simulink model "qless_forgetting_factor_16x16"  (R2021a)
settings: Solver=FixedStepDiscrete  StartTime=0.0  StopTime=stoptime*inf  RelTol=1e-3
InitFcn:
  | qless_init_16chan_fi
undefined symbols (not defined in the file): fc, numArrayElements, physconst, srcAngles, sv, Ts
libraries: hdlsllib x137, commfilt2 x4, commrfcorlib x3, commsync2 x3, commrflib2 x2, commrandsrc3 x2, phasedtxrxlib x2, commdigbbndcpm2 x1, simulink x1, embreciprocals x1, commdigbbndpm3 x1
(part 20 of 22)

== matlab function qless_forgetting_factor_16x16/MVDR_QLess_HDL/Complex Partial-Systolic Matrix Solve Using Q-less QR Decomposition with Forgetting Factor Manually Tiled n=16/Complex Q-less QR Forward Backward Substitute/Complex Burst Back Substitute with Matrix Output1/Reciprocal of the diagonal element/Select diagonal element ==
  data: rIn input; y output; start input; validIn input; validOut output; n parameter
function [y, validOut] = selectDiagonalElement(rIn, start, validIn, n)
%selectDiagonalElement Select diagonal element
%   [y, validOut] = selectDiagonalElement(rIn, start, validIn, m, n)
%   selects a diagonal element from a row of the R matrix, the inverse of
%   which is used in the back substitute computation.
%
%   See also fixed.internal.matrixsolve.selectDiagonalElement.
%
%   Copyright 2019 The MathWorks, Inc.
    
%#codegen

%% INPUTS
% 'rIn' - A non-zero row of the R matrix from the QR decomposition.
%
% 'start' - A boolean signal indicating that a new backsubstitute has
% begun; it thus indicates that new data should be expected.
%
% 'validIn' - A boolean signal indicating that the data on the 'rRow' input
% line is valid.
%
% 'n' (parameter) - The number of columns in the A matrix (and thus rows
% in the R matrix).

%% OUTPUTS
% 'y' - The diagonal element that needs to be inverted.
%
% 'validOut' - A boolean signal indicating that the data on the 'y' output
% line is valid.

%% PERSISTENTS
% 'i' - Counter, and thus tracks which element of the given row needs to be
% inverted. It it initialized to 'numRows' and counts backwards.
%
% 'started' - Indicates if a computation has begun.
persistent i started;

%% CONSTANTS
% 'initialValue', 'finalValue', 'incr' - Constants that help us control the
% behavior of the state machine that selects diagonal elements. If
% 'initialValue' is less than 'finalValue', then the machine is expected to
% perform forward-substitution, and 'incr' should be set to 1. If
% vice-versa, then back-substitution will be performed and 'incr' should be
% set to -1.
initialValue = int16(coder.const(n));
finalValue   = int16(coder.const(1));
incr         = int16(coder.const(-1));

%% MAIN LOOP
if isempty(i)
    % Default persistents. 
    i        = initialValue;
    started  = false;
end

[y,...              % Outputs
 validOut,...
 i,...              % Persistents
 started] = ...  
 fixed.internal.matrixsolve.selectDiagonalElement(rIn,...          % Inputs
                                                  start,...
                                                  validIn,...
                                                  initialValue,... % Constants
                                                  finalValue,...
                                                  incr,...
                                                  i,...            % Persistents 
                                                  started);                       

end

== matlab function qless_forgetting_factor_16x16/MVDR_QLess_HDL/Complex Partial-Systolic Matrix Solve Using Q-less QR Decomposition with Forgetting Factor Manually Tiled n=16/Complex Q-less QR Forward Backward Substitute/Complex Burst Forward Substitute with Matrix Output/Forward substitute logic/Forward substitute state machine ==
  settings: fimath=hdlfimath
  data: rowToSubtract1 output size=[1 p]; rowToSubtract2 output size=[1 p]; inverseElement input size=1; inverseShift input size=1; rIn input size=[1 n]; cIn input size=[1 p]; validIn input boolean size=1; start input boolean size=1; restart input boolean size=1; subtractedRow input size=[1 p]; addedRow input size=[1 p]; multipliedRow input size=[1 p]; finalMultipliedRow input size=[1 p]; rowToAdd1 output size=[1 p]; rowToAdd2 output size=[1 p]; rowToMultiply output size=[1 p]; rElement output size=1; finalRowToMultiply output size=[1 p]; reciprocal output size=1; shiftValue output size=1; xMatrix output size=[n p]; ready output boolean size=1; rowReady output boolean size=1; validOut output boolean size=1; n parameter size=1; p parameter size=1
function [rowToSubtract1,...
          rowToSubtract2,...
          rowToAdd1,...
          rowToAdd2,...
          rowToMultiply,...
          rElement,...
          finalRowToMultiply,...
          reciprocal,...
          shiftValue,...
          xMatrix,...
          ready,...
          rowReady,...
          validOut] = forwardsubStateMachine(inverseElement,...
                                          inverseShift,...
                                          rIn,...
                                          cIn,...
                                          validIn,...
                                          start,...
                                          restart,...
                                          subtractedRow,...
                                          addedRow,...
                                          multipliedRow,...
                                          finalMultipliedRow,...
                                          n,...
                                          p)
%forwardsubStateMachine Implements a state machine that manages the back
%substitute computation to compute the output matrix.
%
%   See also fixed.internal.matrixsolve.selectDiagonalElement.
%
%   Copyright 2019 The MathWorks, Inc.
%#codegen

%% INPUTS
% 'inverseElement' - The reciprocal of the diagonal element to be used
% later.
%
% 'inverseShift' - The reciprocal of the diagonal element is normalized,
% and needs to be denormalized later to yield the correct value.
%
% 'rIn' - A non-zero row of the R matrix from the QR decomposition.
%
% 'cIn' - A row of the Q'B matrix, where Q is obtained from the QR
% decomposition.
%
% 'validIn' - A boolean signal indicating that the data on the input lines
% is valid.
%
% 'start' - A boolean signal indicating that a new backsubstitute has
% begun; it thus indicates that new data should be expected.
%
% 'restart' - A boolean signal to reset the internal state of the block if
% necessary.
%
% 'subtractedRow' - The result of the subraction of the accumulated
% products of the non-diagonal elements of the supplied 'rIn' with the
% rows of the solution matrix, from 'cIn'.
%
% 'addedRow' - The accumulation of the products of the non-diagonal
% elements of the supplied 'rIn' with the rows of the solution matrix.
%
% 'multipliedRow' - The product of a non-diagonal element of the supplied
% 'rIn' with a row from the solution matrix.
%
% 'finalMultipliedRow' - The multiplication of the 'subractedRow' with the
% 'inverseElement' - after shifting by 'inverseShift', this is thus a row
% of the solution matrix.
%
% 'm' (parameter) - The number of rows in A and B matrices.
%
% 'n' (parameter) - The number of columns in the A matrix (and thus rows
% in the R matrix).
%
% 'p' (parameter) - The number of columns in the B matrix (and thus columns
% in the R matrix).

%% OUTPUTS
% 'rowToSubtract1' - This is essentially 'cIn'; we want to subtract the
% accumulated sum (of the products of the non-diagonal elements of 'rIn'
% with the rows of the solution matrix).
%
% 'rowToSubtract2' - This is the accumulated sum of the products of the
%  non-diagonal elements of 'rIn' with the rows of the solution matrix.
%
% 'rowToAdd1' - This is the accumulated sum, so far, of the products of the
%  non-diagonal elements of 'rIn' with the rows of the solution matrix.
%
% 'rowToAdd2' - This is 'multipliedRow' - the product of a non-diagonal
% element of 'rIn' with a row of the solution matrix.
%
% 'rowToMultiply' - A row of the solution matrix - same as 'previousRow'.

% 'rElement' - A non-diagonal element of the supplied 'rIn', to be used to
% multiply with a row of the solution matrix.
%
% 'finalRowToMultiply' - The result of the subraction of the accumulated
% products of the non-diagonal elements of the supplied 'rIn' with the
% rows of the solution matrix, from 'cIn'.
%
% 'reciprocal' - The reciprocal of the diagonal element - same as
% 'inverseElement'.
%
% 'shiftValue' - An integer value used to denormalize the reciprocal - same
% as 'inverseShift'.
%
% 'xMatrix' - The solution to A\B.
%
% 'ready' - A boolean signal indicating the end of computation for the
% entire backsubstitute; it goes high AFTER all the rows of the solution
% matrix have been streamed out.
%
% 'rowReady' - A boolean signal indicating (to the connected logic in the
% hierarchy) that a row of the solution matrix has been computed, and thus
% to signal that the block is ready to accept new data.
%
% 'validOut' - A boolean signal indicating that the data on the output line
% 'outputRow' is valid.

%% PERSISTENTS
% 'mState' - An integer value to hold the state for this FSM. Full
% specifics are listed as comments for each case for this variable.
%
% 'rowCounter' - An integer tracking the row of the solution matrix we are
% currently working on.
%
% 'iterCounter' - An integer tracking which rows of the solution matrix
% have been fetched from the RAM already.
%
% 'sumOfProducts' - The accumulated sum of the products of the non-diagonal
% elements of the supplied 'rIn' with the rows of the solution matrix.
%
% 'finalRowInternal' - Same as finalMultipliedRow.
%
% 'outputMatrix' - The solution to A\B.
%
% 'ramCycleCounter' - An integer counter to track how many cycles have
% passed by since a row of the solution matrix was requested from the RAM.
%
% 'realComplexCycleCounter' - An integer counter to track how many cycles
% have passed by since a real number was multiplied with a complex vector.
%
% 'complexComplexCycleCounter' - An integer counter to track how many
% cycles have passed by since a complex number was multiplied with a
% complex vector.
persistent mState;
persistent rowCounter;
persistent iterCounter;
persistent sumOfProducts;
persistent finalRowInternal;
persistent outputMatrix;
persistent ramCycleCounter;
persistent realComplexCycleCounter;
persistent complexComplexCycleCounter;

%% Get Constants
isComplex = false;
[defaultState,...
    numRows,...
    numColsB,...
    numRamCycles,...
    numRealComplexMulCycles,...
    numComplexComplexMulCycles] = fixed.internal.matrixsolve.getBacksubStateConstants(n,p,isComplex);

%% MAIN LOOP
if isempty(mState)
    % Default persistents.
    mState                      = defaultState;
    rowCounter                  = numRows;
    iterCounter                 = numRows;
    sumOfProducts               = zeros(1, numColsB, 'like', cIn);
    finalRowInternal            = zeros(1, numColsB, 'like', cIn);
    outputMatrix                = zeros(n, p, 'like', cIn);
    ramCycleCounter             = numRamCycles;
    realComplexCycleCounter     = numRealComplexMulCycles;
    complexComplexCycleCounter  = numComplexComplexMulCycles;
end

% [rowToSubtract1,... % Outputs
%  rowToSubtract2,...
%  rowToAdd1,...
%  rowToAdd2,...
%  rowToMultiply,...
%  rElement,...
%  finalRowToMultiply,...
%  reciprocal,...
%  shiftValue,...
%  xMatrix,...
%  ready,...
%  rowReady,...
%  validOut,...
%  mState,...          % Persistents
%  rowCounter,...
%  iterCounter,...
%  sumOfProducts,...
%  finalRowInternal,...
%  ramCycleCounter,...
%  realComplexCycleCounter,...
%  complexComplexCycleCounter] = ...
%  fixed.internal.matrixsolve.forwardsubStateMachineStreamOutMatrix( inverseElement,...  % Inputs
%                                                                 inverseShift,...
%                                                                 rIn,...
%                                                                 cIn,...
%                                                                 validIn,...
%                                                                 start,...
%                                                                 subtractedRow,...
%                                                                 addedRow,...
%                                                                 multipliedRow,...
%                                                                 finalMultipliedRow,...
%                                                                 restart,...
%                                                                 numRows,...         % Constants 
%                                                                 numColsB,...                  
%                                                                 numRamCycles,...                
%                                                                 numRealComplexMulCycles,...
%                                                                 numComplexComplexMulCycles,...
%                                                                 mState,...          % Persistents
%                                                                 rowCounter,...
%                                                                 iterCounter,...
%                                                                 sumOfProducts,...
%                                                                 finalRowInternal,...
%                                                                 outputMatrix,...
%                                                                 ramCycleCounter,...
%                                                                 realComplexCycleCounter,...
%                                                                 complexComplexCycleCounter);

% Describe all possible states.
numStates                   = coder.const(uint8(10));
statesNT                    = numerictype(0, nextpow2(numStates), 0);
defaultState                = fi(0, statesNT);
waitForValidInState         = fi(1, statesNT);
waitForFinalAnswerState     = fi(2, statesNT);
waitForMultiplicationState  = fi(3, statesNT);
waitForAdditionState        = fi(4, statesNT);
waitForSubtractionState     = fi(7, statesNT);

% MAIN LOOP
% NOTE: 'cIn' has the same type as 'previousRow', so they can be used
% interchangeably.

% Default outputs.
rowToSubtract1              = cIn;
rowToSubtract2              = zeros(1, numColsB, 'like', cIn);
rowToAdd1                   = zeros(1, numColsB, 'like', cIn);
rowToAdd2                   = zeros(1, numColsB, 'like', cIn);
rowToMultiply               = zeros(1, numColsB, 'like', cIn);
rElement                    = cast(1, 'like', rIn);
finalRowToMultiply          = cIn;
reciprocal                  = inverseElement;
shiftValue                  = int32(0);
xMatrix                     = zeros(numRows, numColsB, 'like', cIn);
ready                       = false;
rowReady                    = false;
validOut                    = false;

if restart
     % Default persistents.
     isComplex = coder.const(any(~isreal(cIn)));
    [mState,...
    rowCounter,...
    iterCounter,...
    sumOfProducts,...
    finalRowInternal,...
    ramCycleCounter,...
    realComplexCycleCounter,...
    complexComplexCycleCounter] = fixed.internal.matrixsolve.setDefaultPersistentVars(numRows, numColsB, isComplex, cIn);
    outputMatrix = zeros(numRows, numColsB, 'like', cIn);
else
    switch mState
        % STATE 0 - Default case - we end up here at the beginning and
        % the end of each computation, never in between. Wait for 'start'
        % and validIn to go high.
        case defaultState
            % If both 'start' and 'validIn' are high, go to state 2
            % directly and wait for 'finalMultipliedRow'.
            if start && validIn
                rowCounter = numRows;
                mState     = waitForFinalAnswerState;
                % Otherwise, go to state 1 and wait for 'validIn'.
            elseif start
                mState     = waitForValidInState;
                ready      = true;
                % Otherwise, stay here and wait for 'start'/'validIn'.
            else
                mState     = defaultState;
                ready      = true;
            end
            
            % STATE 1 - Wait for 'validIn', but also move to other states
            % depending on some internal variables.
        case waitForValidInState
            % How many iterations do we need?
            iterCounter = numRows;
            
            % Are we done already? Check 'rowCounter' to find out; if yes,
            % stream out the matrix and move to default state.
            if isequal(rowCounter, 0)
                mState          = defaultState;
                ready           = true;
                validOut        = true;
                xMatrix         = outputMatrix;
                rowCounter(:)   = numRows;
                % If this is the first row (from the bottom), then move to
                % state 2 to wait for the final row.
            elseif validIn && isequal(rowCounter, numRows)
                mState          = waitForFinalAnswerState;
                % If not, then multiply previous row with last element of
                % 'rIn'. Then go to state 3, which is the dedicated
                % multiplication state
            elseif validIn
                rowToMultiply   = outputMatrix(numRows, :);
                rElement        = rIn(1);
                mState          = waitForMultiplicationState;
            else
                mState(:)       = waitForValidInState;
            end
            
            % STATE 2 - Wait for 'finalMultipliedRow'.
        case waitForFinalAnswerState
            shiftValue(:)                   = inverseShift;
            finalRowToMultiply              = finalRowInternal;
            % If we get the data on this cycle...
            if isequal(realComplexCycleCounter, 1)
                outputMatrix(rowCounter, :) = finalMultipliedRow;
                % Give values to persistent variables for the next cycle, and set
                % 'rowReady' to high.
                rowReady                    = true;
                mState                      = waitForValidInState;
                realComplexCycleCounter     = numRealComplexMulCycles;
                rowCounter(:)               = rowCounter - 1;
                % ...otherwise, wait here.
            else
                realComplexCycleCounter(:)  = realComplexCycleCounter - 1;
            end
            
            % STATE 3 - Wait for 'multipliedRow'.
        case waitForMultiplicationState
            shiftValue(:)                     = 0;
            % If we get the data on this cycle...
            if isequal(complexComplexCycleCounter, 1)
                % Add the new 'multipliedRow' to the accumulated sum of
                % products so far, and move to state 4.
                rowToAdd1                     = sumOfProducts;
                rowToAdd2                     = multipliedRow;
                mState                        = waitForAdditionState;
                iterCounter(:)                = iterCounter - 1;
                complexComplexCycleCounter    = numComplexComplexMulCycles;
                % ...otherwise, wait here.
            else
                complexComplexCycleCounter(:) = complexComplexCycleCounter - 1;
            end
            
            % STATE 4 - Wait for 'addedRow'. Since addition only takes a single
            % cycle, when we get here we should already have the addition.
        case waitForAdditionState
            sumOfProducts       = addedRow;
            % Now do we go back and do more multiplications, or do we go to
            % subtract the accumulated sum from 'cIn'?
            if isequal(iterCounter, rowCounter)
                rowToSubtract1  = cIn;
                rowToSubtract2  = addedRow;
                mState          = waitForSubtractionState;
            else
                % If iterations are left, fetch more data from the RAM.
                rowToMultiply   = outputMatrix(iterCounter, :);
                rElement        = rIn(numRows + 1 - iterCounter);
                mState          = waitForMultiplicationState;
            end
            
            % STATE 7 - Wait for 'subtractedRow'. Since subtraction only takes
            % a single cycle, when we get here we should already have the
            % subtraction. Then move to state 2 to get 'finalMultipliedRow'.
        case waitForSubtractionState
            reciprocal          = inverseElement;
            finalRowToMultiply  = subtractedRow;
            mState              = waitForFinalAnswerState;
            sumOfProducts       = zeros(1, numColsB, 'like', cIn);
            finalRowInternal    = subtractedRow;
            
            % Catch all other states and go to the default state. Also set all
            % persistent variables to their default values.
        otherwise
            mState                      = defaultState;
            rowCounter                  = numRows;
            iterCounter                 = numRows;
            sumOfProducts               = zeros(1, numColsB, 'like', cIn);
            finalRowInternal            = zeros(1, numColsB, 'like', cIn);
            ramCycleCounter             = numRamCycles;
            realComplexCycleCounter     = numRealComplexMulCycles;
            complexComplexCycleCounter  = numComplexComplexMulCycles;
    end
end


end

== matlab function qless_forgetting_factor_16x16/MVDR_QLess_HDL/Complex Partial-Systolic Matrix Solve Using Q-less QR Decomposition with Forgetting Factor Manually Tiled n=16/Complex Q-less QR Forward Backward Substitute/Complex Burst Forward Substitute with Matrix Output/Forward substitute logic/Variable shift/MATLAB Function ==
  settings: fimath=hdlfimath
  data: x input size=[1 p]; y output size=[1 p]; shiftValue input
function y = fcn(x,shiftValue)
    if isfi(x) && isscaledtype(x)
        y = bitshift(x, shiftValue);
    else
        y = cast(double(x)* 2.^double(shiftValue),'like',x);
    end
end

== matlab function qless_forgetting_factor_16x16/MVDR_QLess_HDL/Complex Partial-Systolic Matrix Solve Using Q-less QR Decomposition with Forgetting Factor Manually Tiled n=16/Complex Q-less QR Forward Backward Substitute/Complex Burst Forward Substitute with Matrix Output/Cast to Union of Types ==
  settings: fimath=hdlfimath
  data: Xref input; Cout output; Cin input
function Cout = castToUnionType(Xref,Cin)
    %castToUnionType Cast second input to union of the two types
    T = fixed.internal.type.unionPrototype(Cin,Xref,...
        'RoundingMethod','Floor',...
        'OverflowAction','Wrap');
    Cout = cast(Cin,'like',T);
end

== matlab function qless_forgetting_factor_16x16/MVDR_QLess_HDL/Complex Partial-Systolic Matrix Solve Using Q-less QR Decomposition with Forgetting Factor Manually Tiled n=16/Complex Q-less QR Forward Backward Substitute/Complex Burst Forward Substitute with Matrix Output/Reciprocal of the diagonal element/Positive Normalized Reciprocal HDL Optimized/Positive Real CORDIC Reciprocal Kernel HDL Optimized/positiveNormalizedCORDICReciprocal ==
  settings: fimath=hdlfimath
  data: x input; t_in input; y output; t output; validIn input; validOut output
function [y, t, validOut] = positiveNormalizedCORDICReciprocal(x, t_in, validIn)
%positiveNormalizedCORDICReciprocal Positive normalized reciprocal
%   [y, t, validOut] = positiveNormalizedCORDICReciprocal(x, t_in, validIn)
%   produces y = 1/x when 1 <= x < 2, and t = t_in.
%
%   When x = 0 and x is fixed-point or scaled-double, then y = 2 - eps(y).
%
%   When x = 0 and x is a floating-point type, then y = inf.
%
%   If x is fixed-point, then y is fixed-point with
%   numerictype(1, x.WordLength, x.WordLength - 2).
%
%   If x is floating-point, then y is floating-point of the same type.
%
%   References:
%
%   [1] Jack E. Volder, "The CORDIC Trigonometric Computing Technique," IRE
%       Transactions on Electronic Computers, Volume EC-8, September 1959,
%       pp. 330-334.
%
%   [2] J.S. Walther, "A Unified Algorithm for Elementary Functions,"
%       Conference Proceedings, Spring Joint Computer Conference, May 1971,
%       pp. 379-385.
%
%   See also fixed.internal.reciprocal.cordicReciprocalKernel.

%   Copyright 2019 The MathWorks, Inc.
%#codegen
    fixed.internal.reciprocal.validateReciprocalInputs(x, validIn);
    if isfi(x) && isscaledtype(x)
        % CORDIC reciprocal for fixed-point and scaled-double types
        [y,t,validOut] = fixedpointReciprocal(x,t_in,validIn);
    else
        % y = 1/x for builtin types.
        y = 1./x;
        t = t_in;
        validOut = validIn;
    end
end

function [reciprocal, t, validOut] = fixedpointReciprocal(xIn,t_in, validIn)
%fixedpointReciprocal Fixed-point reciprocal
%   [reciprocal, t, validOut] = fixedpointReciprocal(xIn, t_in, validIn)
%   Given real scalar xIn such that 1 <= xIn < 2 this function produces
%   reciprocal such that
%
%      reciprocal = 1/xIn.
%
%   and reciprocal is in the range 0.5 < reciprocal <= 1.
%
%   When xIn = 0, then y = 2 - eps(y).
%
%   The input is only valid when validIn = true.  The output is only
%   valid when validOut = true.
%
%   The output t is identical to t_in, synchronized by validIn/validOut.
    [T,NumberOfCordicIterations] = fixed.internal.reciprocal.positiveReciprocalTypes(xIn);
    % Register variables for the CORDIC Reciprocal Kernel
    persistent xReg yReg zReg validReg tReg
    if isempty(xReg)
        xReg = zeros(NumberOfCordicIterations+2,1,'like',T.x);
        yReg = zeros(NumberOfCordicIterations+2,1,'like',T.x);
        zReg = zeros(NumberOfCordicIterations+2,1,'like',T.x);
        validReg = zeros(NumberOfCordicIterations+2,1,'like',validIn);
        tReg = zeros(NumberOfCordicIterations+2,1,'like',t_in);
    end
    % CORDIC Reciprocal Kernel
    [reciprocal,t,validOut,...
        xReg,yReg,zReg,validReg,tReg... % Persistent variables
        ] = fixed.internal.reciprocal.cordicReciprocalKernel(xIn,t_in,validIn,...
        xReg,yReg,zReg,validReg,tReg... % Persistent variables
        );
end

== matlab function qless_forgetting_factor_16x16/MVDR_QLess_HDL/MATLAB Function ==
  data: write_en output; valid_i input; isEmpty input; qr_ready input; read_en output
function [write_en, read_en]= amat_scheduler(valid_i, isEmpty, qr_ready)
persistent scheduler_state counter

STATE_IS_LOADING_MAT = fi(0,0,4,0);
WAIT_FOR_SOLVE = fi(1,0,4,0);
MAX_FIFO_DEPTH = 16;
if isempty(scheduler_state)
    scheduler_state = STATE_IS_LOADING_MAT;
    counter = uint32(0);
end

write_en = false;
read_en = false;
switch(scheduler_state)
    case(STATE_IS_LOADING_MAT)
        if valid_i
            if counter < MAX_FIFO_DEPTH
                write_en = true;
                counter(:) = counter + 1;
            else
                scheduler_state(:) = WAIT_FOR_SOLVE;
                counter(:) = 0;            
            end            
        end
    case(WAIT_FOR_SOLVE)
        if qr_ready
            if counter < MAX_FIFO_DEPTH
                read_en = true;
                counter(:) = counter + 1; 
            else
                scheduler_state(:) = STATE_IS_LOADING_MAT;
                counter(:) = 0;         
            end
        end
       
end



%  if isEmpty
%             scheduler_state(:) = STATE_IS_LOADING_MAT;
%         else
%             if qr_ready
%                 read_en = true;
%             end
%  end
%         
 
% if ~isEmpty && qr_ready
%     read_en = true;
% end


end

== matlab function qless_forgetting_factor_16x16/MVDR_QLess_HDL/Complex Partial-Systolic Matrix Solve Using Q-less QR Decomposition with Forgetting Factor Manually Tiled n=16/Complex Q-less QR Forward Backward Substitute/Complex Burst Forward Substitute with Matrix Output/Reciprocal of the diagonal element/Positive Normalized Reciprocal HDL Optimized/Positive Real Normalizer HDL Optimized/positiveRealNormalizer ==
  settings: fimath=hdlfimath
  data: u input; x output; validIn input; e output; validOut output
function [x, e, validOut] = positiveRealNormalizer(u, validIn)
%positiveRealNormalizer  Positive real normalizer
%   [x, e, validOut] = positiveRealNormalizer(u, validIn) produces
%   x such that 1 <= x < 2 and e such that x = (2^e)*u when u > 0.
%
%   When u = 0 and u is fixed-point or scaled-double, then x = 0 and
%   e = (2^nextpow2(x.WordLength)) - x.WordLength - x.FractionLength.
%
%   When u = 0 and u is floating-point, then x = 0 and e = 1.
%
%   See also fixed.internal.reciprocal.normalizePositiveFixedPoint,
%   fixed.internal.reciprocal.normalizePositiveFloatOrScaledDouble.

%   Copyright 2019 The MathWorks, Inc.
%#codegen

% This function only works on scalars.
% Only operate on the real part
    fixed.internal.reciprocal.validateNormalizerInputs(u, validIn);
    % Normalize in unsigned type.
    [x_normalized, n_normalized, validOut] = normalize(real(u), validIn);
    % Cast the output to signed if the input was signed.
    x = fixed.internal.reciprocal.castToInputSignedness(x_normalized,u);
    % Convert the normalized shift value based on the data type of the
    % input U so that the output of the normalizer X is in real-world
    % scale and X = (2^N)*U.
    e = fi(int32(0));
    e(:) = fixed.internal.reciprocal.normalizedShiftToRealWorldValueShift(n_normalized,u);
end

function [x_normalized, e_normalized, validOut] = normalize(u, validIn)
    if isfi(u) && isfixed(u)
        % Normalize fixed-point values
        [x_normalized, e_normalized,validOut] = normalizeFixedpoint(u, validIn);
    else
        % Normalize floating-point or scaled-double
        [x_normalized, e_normalized, validOut] = fixed.internal.reciprocal.normalizePositiveFloatOrScaledDouble(u, validIn);
    end
end

function [u_normalized, e_normalized,validOut] = normalizeFixedpoint(u, validIn)
% Normalize fixed-point values.
    persistent validReg
    persistent tReg
    persistent xReg
    % For fixed-point types, the normalization uses a binary search of
    % length log2 of the word length of the input.
    number_of_stages = coder.const(nextpow2(u.WordLength));

    if isempty(validReg)
        validReg = false(number_of_stages+1,1);
        tReg = zeros(number_of_stages+1,1,'like',fi(0,0,max(number_of_stages,1),0));
        xReg = zeros(number_of_stages+1,1,'like',fi([],0,u.WordLength,0));
    end

    [u_normalized, e_normalized,validOut,...
        validReg, tReg,xReg...  % Persistent
        ] = fixed.internal.reciprocal.normalizePositiveFixedPoint(u, validIn, number_of_stages, ...
        validReg, tReg,xReg...  % Persistent
        );
end

== matlab function qless_forgetting_factor_16x16/MVDR_QLess_HDL/Complex Partial-Systolic Matrix Solve Using Q-less QR Decomposition with Forgetting Factor Manually Tiled n=16/Complex Q-less QR Forward Backward Substitute/Complex Burst Forward Substitute with Matrix Output/Reciprocal of the diagonal element/Select diagonal element ==
  data: rIn input; y output; start input; validIn input; validOut output; n parameter
function [y, validOut] = selectDiagonalElement(rIn, start, validIn, n)
%selectDiagonalElement Select diagonal element
%   [y, validOut] = selectDiagonalElement(rIn, start, validIn, m, n)
%   selects a diagonal element from a row of the R matrix, the inverse of
%   which is used in the back substitute computation.
%
%   See also fixed.internal.matrixsolve.selectDiagonalElement.
%
%   Copyright 2019 The MathWorks, Inc.
    
%#codegen

%% INPUTS
% 'rIn' - A non-zero row of the R matrix from the QR decomposition.
%
% 'start' - A boolean signal indicating that a new backsubstitute has
% begun; it thus indicates that new data should be expected.
%
% 'validIn' - A boolean signal indicating that the data on the 'rRow' input
% line is valid.
%
% 'n' (parameter) - The number of columns in the A matrix (and thus rows
% in the R matrix).

%% OUTPUTS
% 'y' - The diagonal element that needs to be inverted.
%
% 'validOut' - A boolean signal indicating that the data on the 'y' output
% line is valid.

%% PERSISTENTS
% 'i' - Counter, and thus tracks which element of the given row needs to be
% inverted. It it initialized to 'numRows' and counts backwards.
%
% 'started' - Indicates if a computation has begun.
persistent i started;

%% CONSTANTS
% 'initialValue', 'finalValue', 'incr' - Constants that help us control the
% behavior of the state machine that selects diagonal elements. If
% 'initialValue' is less than 'finalValue', then the machine is expected to
% perform forward-substitution, and 'incr' should be set to 1. If
% vice-versa, then back-substitution will be performed and 'incr' should be
% set to -1.
initialValue = int16(coder.const(1));
finalValue   = int16(coder.const(n));
incr         = int16(coder.const(1));

%% MAIN LOOP
if isempty(i)
    % Default persistents. 
    i        = initialValue;
    started  = false;
end

[y,...              % Outputs
 validOut,...
 i,...              % Persistents
 started] = ...  
 fixed.internal.matrixsolve.selectDiagonalElement(rIn,...          % Inputs
                                                  start,...
                                                  validIn,...
                                                  initialValue,... % Constants
                                                  finalValue,...
                                                  incr,...
                                                  i,...            % Persistents 
                                                  started);                       

end

== matlab function qless_forgetting_factor_16x16/MVDR_QLess_HDL/Complex Partial-Systolic Matrix Solve Using Q-less QR Decomposition with Forgetting Factor Manually Tiled n=16/Complex Q-less QR Forward Backward Substitute/Partial-Systolic Matrix Solve Q-less QR B Buffer Manager/B Buffer Manager State Machine ==
  data: rowForFwdSub input; Lrow output; fwdSubValidIn input size=1; bValidIn input size=1; backSubDone input size=1; restart input boolean size=1; rowIndex output fixdt('uint32', 'DataTypeOverride', 'Off') size=1; validOut output boolean size=1; start output boolean size=1; readyForFwdSub output boolean size=1; n parameter size=1
function [Lrow,...
        rowIndex,...
        validOut,...
        start,...
        readyForFwdSub] = ...
        manageBufferForBStateMachine(...
        rowForFwdSub,...
        fwdSubValidIn,...
        bValidIn,...
        backSubDone,...
        restart,...
        n)
    
    % State names
    DEFAULT = uint8(0);
    STARTFORWARDSUBSTITUTE = uint8(1);
    MANAGEFORWARDSUBSTITUTE = uint8(2);
    FINISHFORWARDSUBSTITUTE = uint8(3);
    
    persistent mState
    persistent mRowIndex
    persistent mValidOut
    persistent mStart
    persistent mLrow
    persistent mReadyForFwdSub
    
    % Init persistents.
    if isempty(mState)
        mState = DEFAULT;
        mRowIndex = uint32(1);
        mValidOut = false;
        mStart = false;
        mLrow = zeros(size(rowForFwdSub),'like',rowForFwdSub);
        mReadyForFwdSub = false;
    end
    state = mState;
    rowIndex = mRowIndex;
    validOut = mValidOut;
    start = mStart;
    Lrow = mLrow;
    readyForFwdSub = mReadyForFwdSub;
    if restart
        % If 'restart' is high, re-initialize everything.
        mState = DEFAULT;
        mLrow = rowForFwdSub;
        mRowIndex(:) = 1;
        mValidOut = false;
        mStart = false;
        mReadyForFwdSub = false;
    else
        % Otherwise, enter the main loop.
        mLrow = rowForFwdSub;
        mValidOut = false;
        mStart = false;
        mReadyForFwdSub = false;
        switch state
            case DEFAULT
                % Default state: accept the incoming B matrix when validIn is high,
                % and then move on to the next state.
                if bValidIn
                    mRowIndex(:) = 1;
                    mState(:) = STARTFORWARDSUBSTITUTE;
                    mStart = true;
                    mReadyForFwdSub = true;
                else
                end
                
            case STARTFORWARDSUBSTITUTE
                % Start the forward substitute (i.e., send one
                % row), and then move on to MANAGEFORWARDSUBSTITUTE.
                mReadyForFwdSub = true;
                if fwdSubValidIn
                    mLrow = rowForFwdSub;
                    mValidOut = true;
                    mState(:) = MANAGEFORWARDSUBSTITUTE;
                end
                
            case MANAGEFORWARDSUBSTITUTE
                % Manage the forward substitute. Send a new row from the B
                % matrix when it's needed. At the end, move to
                % FINISHFORWARDSUBSTITUTE.
                if fwdSubValidIn && ~isequal(mRowIndex, n)
                    mRowIndex(:) = mRowIndex + 1;
                    mValidOut = true;
                elseif isequal(mRowIndex, n)
                    mState(:)= FINISHFORWARDSUBSTITUTE;
                else
                end
                
            case FINISHFORWARDSUBSTITUTE
                % Wait for the back substitute to end; then wait to receive
                % another B matrix.
                if backSubDone
                    mState(:) = DEFAULT;
                    mRowIndex(:) = 1;
                end
        end
    end
    
end

== matlab function qless_forgetting_factor_16x16/MVDR_QLess_HDL/Complex Partial-Systolic Matrix Solve Using Q-less QR Decomposition with Forgetting Factor Manually Tiled n=16/Complex Q-less QR Forward Backward Substitute/Partial-Systolic Matrix Solve Q-less QR B Buffer Manager/Save Matrix B/Enabled Delay ==
  data: dataIn input; dataOut output; writeEnable input; restart input
function dataOut = enabledDelay(dataIn,writeEnable,restart)
    persistent mData
    if isempty(mData)
        mData = zeros(size(dataIn),'like',dataIn);
    end
    dataOut = mData;
    if restart
        mData = zeros(size(dataIn),'like',dataIn);
    elseif writeEnable
        mData = dataIn;
    end
end

== matlab function qless_forgetting_factor_16x16/MVDR_QLess_HDL/Complex Partial-Systolic Matrix Solve Using Q-less QR Decomposition with Forgetting Factor Manually Tiled n=16/Complex Q-less QR Forward Backward Substitute/Partial-Systolic Matrix Solve Q-less QR Forward Substitute Memory Manager/MATLAB Function1 ==
  data: rowIndex output fixdt('uint32', 'DataTypeOverride', 'Off') size=1; inputValidIn input; needFwdSubRow input; backSubDone input; restart input; validOut output; needBackSubRow output; n parameter size=1
function [...
        rowIndex,...
        validOut,...
        needBackSubRow] = ...
        fwdSubBuffer(...
        inputValidIn,...
        needFwdSubRow,...
        backSubDone,...
        restart,...
        n)

    % State names
    DEFAULT = uint8(0);
    STARTBACKWARDSUBSTITUTE = uint8(1);
    MANAGEBACKWARDSUBSTITUTE = uint8(2);
    FINISHBACKWARDSUBSTITUTE = uint8(3);

    persistent mRowIndex;
    persistent mState;
    
    % Initialize persistents.
    if isempty(mState)
        mRowIndex = uint32(1);
        mState = DEFAULT;
    end
    
    rowIndex = mRowIndex;
    
    if restart
        % If 'restart' is high, re-initialize everything.
        mRowIndex(:) = 1;
        mState(:) = DEFAULT;
        validOut  = false;
        needBackSubRow = false;
    else
        % Otherwise, enter the main loop.
        validOut  = false;
        needBackSubRow = false;
        switch mState
            case DEFAULT
                % Default state: Accept the output of the forward
                % substitute. Once n rows have been received, move to state
                % STARTFORWARDSUBSTITUTE.
                if inputValidIn
                    mState(:) = STARTBACKWARDSUBSTITUTE;
                    mRowIndex(:) = 1;
                else
                end
                
            case STARTBACKWARDSUBSTITUTE
                % Start the backward substitute (i.e., send a single row)
                % and then move to state MANAGEBACKWARDSUBSTITUTE.
                mRowIndex(:) = 1;
                validOut  = true;
                needBackSubRow = true;
                mState(:) = MANAGEBACKWARDSUBSTITUTE;
                
            case MANAGEBACKWARDSUBSTITUTE
                % Manage the backward substitute. Send a new row from the
                % assembled matrix when it's needed. At the end, move to
                % state FINISHBACKWARDSUBSTITUTE.
                if needFwdSubRow && ~isequal(mRowIndex, n)
                    mRowIndex(:) = mRowIndex + 1;
                    validOut  = true;
                    needBackSubRow = true;
                elseif isequal(mRowIndex, n)
                    mState(:) = FINISHBACKWARDSUBSTITUTE;
                else
                end
                
            case FINISHBACKWARDSUBSTITUTE
                % Wait for the backward substitute to end; then move on to
                % the default state.
                if backSubDone
                    mState(:) = DEFAULT;
                    mRowIndex(:) = 1;
                end
        end
    end
end

== matlab function qless_forgetting_factor_16x16/MVDR_QLess_HDL/Complex Partial-Systolic Matrix Solve Using Q-less QR Decomposition with Forgetting Factor Manually Tiled n=16/Complex Q-less QR Forward Backward Substitute/Partial-Systolic Matrix Solve Q-less QR Forward Substitute Memory Manager/Save Matrix B/Enabled Delay ==
  data: dataIn input; dataOut output; writeEnable input; restart input
function dataOut = enabledDelay(dataIn,writeEnable,restart)
    persistent mData
    if isempty(mData)
        mData = zeros(size(dataIn),'like',dataIn);
    end
    dataOut = mData;
    if restart
        mData = zeros(size(dataIn),'like',dataIn);
    elseif writeEnable
        mData = dataIn;
    end
end

== matlab function qless_forgetting_factor_16x16/MVDR_QLess_HDL/Complex Partial-Systolic Matrix Solve Using Q-less QR Decomposition with Forgetting Factor Manually Tiled n=16/Complex Q-less QR Forward Backward Substitute/Partial-Systolic Matrix Solve Q-less QR Output Manager/Partial-Systolic Manage QR Output State Machine ==
  data: validIn input size=1; columnOutIndex output fixdt('uint32', 'DataTypeOverride', 'Off') size=1; needRowFwdSub input size=1; needRowBackSub input size=1; backSubDone input size=1; restartIn input size=1; readyForFwdSub input size=1; fwdSubValidOut output size=1; rowOutIndex output fixdt('uint32', 'DataTypeOverride', 'Off') size=1; n parameter size=1; validR output size=1; restartOut output size=1
function [columnOutIndex,...
        fwdSubValidOut,...
        rowOutIndex,...
        validR,...
        restartOut] = manageQlessOutput(...
        validIn,...
        needRowFwdSub,...
        needRowBackSub,...
        backSubDone,...
        restartIn,...
        readyForFwdSub,...
        n)
    
    % State names
    DEFAULT = uint8(0);
    START = uint8(7);
    FORWARDSUBSTITUTE = uint8(1);
    STARTBACKWARDSUBSTITUTE = uint8(2);
    BACKWARDSUBSTITUTE = uint8(3);
    ENDBACKWARDSUBSTITUTE = uint8(4);
    WAITFORBMATRIX = uint8(5);
    CONTINUEFORWARDSUBSTITUTE = uint8(8);
    BMATRIXREADY = uint8(6);
    
    % Initial output values
    columnOutIndex = uint32(1);
    fwdSubValidOut = false;
    rowOutIndex = uint32(1);
    validR = false;
    restartOut = false;
    
    % persistent r;
    persistent i;
    persistent mState;
    
    % Init persistents.
    if isempty(mState)
        i              = uint32(n);
        mState         = DEFAULT;
    end
    
    
    % If 'restart' is high, re-initialize everything.
    if restartIn
        restartOut = true;
        rowOutIndex(:) = n;
        columnOutIndex(:) = n;
        i(:)           = n;
        mState(:)      = DEFAULT;
    else
        % Otherwise, enter the main loop.
        rowOutIndex(:) = i;
        columnOutIndex(:) = i;
        switch mState
            % Default state: Wait for validIn (the validOut of the previous
            % block) to go high 'n' times, where 'n' is the number of columns
            % in the A matrix. Once validIn goes high 'n' times, 'start' the
            % forward substitution process and move to state FORWARDSUBSTITUTE.
            case DEFAULT
                if validIn
                    validR = true;
                    mState(:) = START;
                    fwdSubValidOut = false;
                    i(:) = 1;
                else
                end
                
            case START
                fwdSubValidOut = true;
                columnOutIndex(:) = 1;
                i(:) = 1;
                mState = FORWARDSUBSTITUTE;
                
                % Manage the forward sub. Whenever 'needRowFwdSub'
                % goes high, send a new column of the R matrix. Once all columns
                % are sent, move to state STARTBACKWARDSUBSTITUTE.
            case FORWARDSUBSTITUTE
                if needRowFwdSub && ~isequal(i, n)
                    columnOutIndex(:) = i + 1;
                    i(:)           = i + 1;
                    fwdSubValidOut = true;
                elseif isequal(i, n)
                    mState(:)      = STARTBACKWARDSUBSTITUTE;
                else
                end
                
                % Start the back sub (i.e., send the first row), and then
                % move on to state BACKWARDSUBSTITUTE.
            case STARTBACKWARDSUBSTITUTE
                if needRowBackSub && isequal(i, n)
                    rowOutIndex(:) = i;
                    mState(:)     = BACKWARDSUBSTITUTE;
                end
                
                % Manage the back sub. Send a new row from the R matrix
                % when it's needed. At the end, move to state ENDBACKWARDSUBSTITUTE.
            case BACKWARDSUBSTITUTE
                if needRowBackSub && ~isequal(i, 1)
                    rowOutIndex(:) = i - 1;
                    i(:)          = i - 1;
                elseif isequal(i, 1)
                    mState(:) = ENDBACKWARDSUBSTITUTE;
                else
                end
                
                % Wait for the back sub to end; then move on to the
                % state where we wait for the B matrix to be ready before accepting
                % the new R matrix.
            case ENDBACKWARDSUBSTITUTE
                if backSubDone
                    mState(:) = WAITFORBMATRIX;
                    i(:)      = n;
                end
                
                % Wait for the B matrix to be ready. If it is, accept the
                % data when validIn goes high and use it. If it is, just move on to
                % the next intermediate state that will wait for B before sending
                % it out. The reason for having an extra state is that we need to
                % be sure that we have the latest data when B is ready. If we hold
                % on to the data we receive in this state (when validIn goes high),
                % then by the time B is assembled/ready the data might be old.
            case WAITFORBMATRIX
                if validIn && readyForFwdSub
                    fwdSubValidOut = false;
                    validR = true;
                    i(:) = 1;
                    mState(:) = CONTINUEFORWARDSUBSTITUTE;
                elseif validIn
                    mState(:) = BMATRIXREADY;
                else
                end
                
            case CONTINUEFORWARDSUBSTITUTE
                fwdSubValidOut = true;
                columnOutIndex(:) = 1;
                i(:) = 1;
                mState(:) = FORWARDSUBSTITUTE;
                
            case BMATRIXREADY
                if readyForFwdSub
                    mState(:) = FORWARDSUBSTITUTE;
                    fwdSubValidOut = true;
                    columnOutIndex(:) = 1;
                    i(:) = 1;
                end
        end
    end
    
end

== matlab function qless_forgetting_factor_16x16/MVDR_QLess_HDL/Complex Partial-Systolic Matrix Solve Using Q-less QR Decomposition with Forgetting Factor Manually Tiled n=16/Complex Partial-Systolic Q-less QR with Forgetting Factor/Complex Partial-Systolic Q-less QR with Forgetting Factor Manually tiled/Complex Partial-Systolic Q-less QR Decomposition with Forgetting Factor Section Constant pivot11/Complex Partial-Systolic Q-less QR Row Rotations/Q-less QR Rotate First Element To Real1/Q-less QR Real Row Rotations/Inverse CORDIC Gain1/MATLAB Function ==
  data: u input; y output
function y = inverseCORDICGain(u)
    %inverseCORDICGain Multiply by the inverse of the CORDIC gain constant
    %   Y = inverseCORDICGain(U) multiplies input U by the inverse CORDIC
    %   gain constant.  The data type of output Y is the same as the data
    %   type of input U.  This data type will never overflow because the
    %   inverse CORDIC gain constant quickly converges to around 0.60725 as
    %   a function of the word length of the input.
    F = fixed.fimathLike(u);
    [~, Kn] = fixed.cordicConstants(u);
    y = setfimath(u,F) * Kn;
end
